simulink model "complex_closed"  (Simulink 6.0)
settings: Solver=ode3  StartTime=0.0  StopTime=10.0  FixedStep=0.01  RelTol=1e-3
settings Model: LastModifiedBy=Administrator

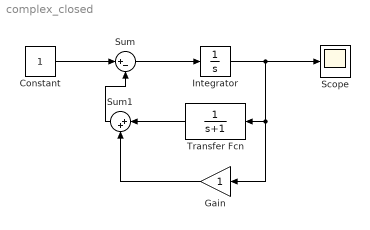
== system complex_closed ==
  Constant : Constant
  Gain : Gain  Orientation=left
  Integrator : Integrator
  Scope : Scope
      settings: SaveName=out  DataFormat=Array
  Sum : Sum  Inputs=|+-
  Sum1 : Sum  Orientation=left  Inputs=|++
  Transfer Fcn : TransferFcn  Orientation=left  Denominator=[1 1]
  wires:
  Integrator/1 -> Scope/1, Transfer Fcn/1, Gain/1
  Constant/1 -> Sum/1
  Sum/1 -> Integrator/1
  Gain/1 -> Sum1/2
  Transfer Fcn/1 -> Sum1/1
  Sum1/1 -> Sum/2
